simulink model "Car24withDspace"  (R2024a)
settings: Solver=FixedStepAuto  StartTime=0.0  StopTime=Inf  FixedStep=0.001  RelTol=1e-3
PostLoadFcn:
  | if any(exist('dsrtsu_mdlpostloadfcn', 'file') ~= 0), dsrtsu_mdlpostloadfcn('Execute', bdroot); end
InitFcn:
  | , if any(exist('dsmpb_private', 'file') ~= 0), dsmpb_private('dsmpb_mdlclblib', 'Init', bdroot); end,
model workspace (MAT data in the model file):
  indicator = -1
libraries: dsmpblib x8
PreSaveFcn:
  | , if any(exist('dsmpb_private', 'file') ~= 0), dsmpb_private('dsmpb_mdlclblib', 'PreSave', bdroot); end,
CloseFcn:
  | , if any(exist('dsmpb_private', 'file') ~= 0), dsmpb_private('dsmpb_mdlclblib', 'Close', bdroot); end,
settings Model: DSMPB_ID_DATA={'798',struct('BlockId','ba278ee5-6691-4485-94d8-efd942a21a20','SignalIds',{{'fcd8faac-c2ce-41ea-aead-0dfdf2c47ef0'}}),'799',struct('BlockId','a8e41c90-77fc-4f06-b46f-94a13d6c991a','SignalIds',{{'22f08aa9-6fcd-41a1-b62d-e962f18854da'}}),'800',struct('BlockId','31fcda0f-fd6e-4941-ae8a-2ba19cb6e7f7','SignalIds',{{'35c98d34-17e7-4115-963b-beec5af4cec8'}}),'801',struct('BlockId','201071ae-2b6e-446e-b4ec-6a6734ee09dc','SignalIds',{{'1d100d76-8f1b-4c24-9a3c-279a1ced5831'}}),'802',struct('BlockId','a6d9fb5c-79d9-4b84-be40-f4d025ad3cea','SignalIds',{{'1cd988e0-b042-4718-91dc-4e913c3a45d9'}}),'803',struct('BlockId','53d4ca67-4f96-4e4a-b985-d2b7837ee7a0','SignalIds',{{'230ce85a-856b-4b55-a826-97e40144e857'}}),'804',struct('BlockId','a190365b-236b-46d3-8d77-caf955faebcf','SignalIds',{{'146f610b-4436-47f4-bba7-306650b5bba2'}}),'805',struct('BlockId','8fdb49cd-8d95-41ce-94e1-bab524caa5ea','SignalIds',{{'c30a0cdc-fc87-413d-a2e7-a08f688cb26a'}})}  Creator=thipp  LastModifiedBy=thipp
settings SolverCC: AutoInsertRateTranBlk=on
settings OptimizationCC: BlockReduction=off  ConditionallyExecuteInputs=off  OptimizeBlockIOStorage=off  BufferReuse=off  EnhancedBackFolding=on  PassReuseOutputArgsThreshold=0  MaxStackSize=64  OptimizeBlockOrder=speed  DifferentSizesBufferReuse=on
settings DebuggingCC: TasksWithSamePriorityMsg=none  ParameterTunabilityLossMsg=error
settings HardwareCC: ProdBitPerLong=64  ProdLargestAtomicInteger=Integer  ProdWordSize=32  ProdLongLongMode=on  ProdHWDeviceType=Custom Processor->Custom  UseEmbeddedCoderFeatures=off  UseSimulinkCoderFeatures=off
settings ModelReferenceCC: EnableParallelModelReferenceBuilds=on
settings SFSimCC: MATLABDynamicMemAlloc=off
settings RTWCC: Description=dSPACE Target DSRT - Generates SIC files for import by ConfigurationDesk and VEOS. Provides code generation for Simulink models imported in ConfigurationDesk.  SystemTargetFile=dsrt.tlc  GenCodeOnly=on  MakeCommand=make_dsrt  TemplateMakefile=dsrt_default_tmf  RTWVerbose=off  BuildConfiguration=Faster Runs
settings CodeAppCC: ForceParamTrailComments=on  OperatorAnnotations=on
settings STFCustomTargetCC: TargetLangStandard=C89/C90 (ANSI)  ParMdlRefBuildCompliant=on  GRTInterface=off  UseToolchainInfoCompliant=off  SystemTargetFile=dsrt.tlc
settings GRTTargetCC: TargetLangStandard=C89/C90 (ANSI)  CompOptLevelCompliant=off  ConcurrentExecutionCompliant=off  CombineOutputUpdateFcns=off  MatFileLogging=off  CPPClassGenCompliant=off  UseToolchainInfoCompliant=off

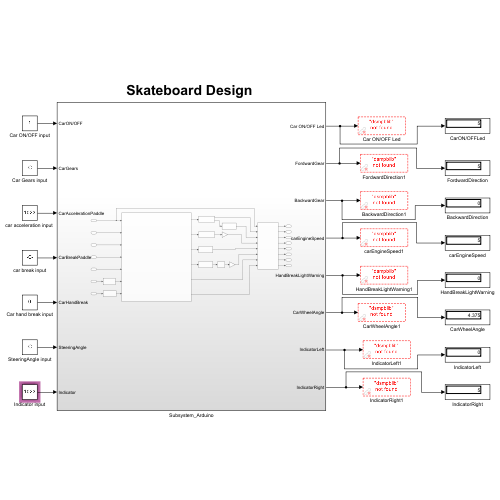
[thumbnail: Simulink's stored preview of the top-level diagram]
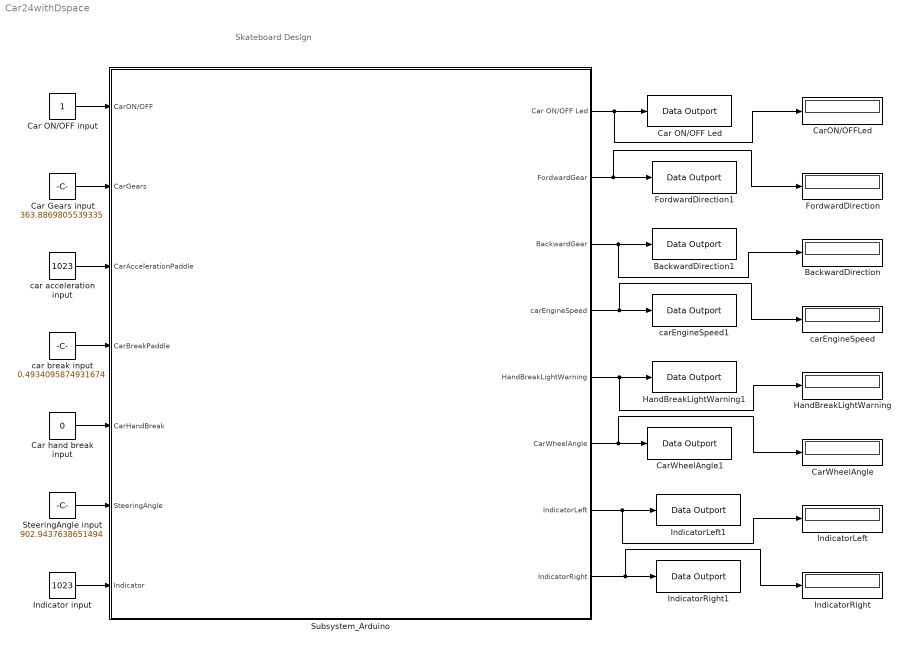
== system Car24withDspace ==
  note: Skateboard Design
  BackwardDirection : Display
  BackwardDirection1 : dsmpblib/Data Outport  Priority=-10000
      settings: SourceProductName=dSPACE Model Interface Package for Simulink (MIPS)
  Car Gears input : Constant  Value=363.8869805539335
  Car ON/OFF Led : dsmpblib/Data Outport  Priority=-10000
      settings: SourceProductName=dSPACE Model Interface Package for Simulink (MIPS)
  Car ON/OFF input : Constant
  Car hand break input : Constant  Value=0
  CarON/OFFLed : Display
  CarWheelAngle : Display
  CarWheelAngle1 : dsmpblib/Data Outport  Priority=-10000
      settings: SourceProductName=dSPACE Model Interface Package for Simulink (MIPS)
  FordwardDirection : Display
  FordwardDirection1 : dsmpblib/Data Outport  Priority=-10000
      settings: SourceProductName=dSPACE Model Interface Package for Simulink (MIPS)
  HandBreakLightWarning : Display
  HandBreakLightWarning1 : dsmpblib/Data Outport  Priority=-10000
      settings: SourceProductName=dSPACE Model Interface Package for Simulink (MIPS)
  Indicator input : Constant  Value=1023
  IndicatorLeft : Display
  IndicatorLeft1 : dsmpblib/Data Outport  Priority=-10000
      settings: SourceProductName=dSPACE Model Interface Package for Simulink (MIPS)
  IndicatorRight : Display
  IndicatorRight1 : dsmpblib/Data Outport  Priority=-10000
      settings: SourceProductName=dSPACE Model Interface Package for Simulink (MIPS)
  SteeringAngle input : Constant  Value=902.9437638651494
  Subsystem_Arduino : Subsystem
  "car acceleration input " : Constant  Value=1023
  car break input : Constant  Value=0.4934095874931674
  carEngineSpeed : Display
  carEngineSpeed1 : dsmpblib/Data Outport  Priority=-10000
      settings: SourceProductName=dSPACE Model Interface Package for Simulink (MIPS)
  wires:
  Subsystem_Arduino/3(BackwardGear) -> BackwardDirection1/1, BackwardDirection/1
  Subsystem_Arduino/4(carEngineSpeed) -> carEngineSpeed1/1, carEngineSpeed/1
  Subsystem_Arduino/5(HandBreakLightWarning) -> HandBreakLightWarning1/1, HandBreakLightWarning/1
  Subsystem_Arduino/6(CarWheelAngle) -> CarWheelAngle1/1, CarWheelAngle/1
  Subsystem_Arduino/7(IndicatorLeft) -> IndicatorLeft1/1, IndicatorLeft/1
  Subsystem_Arduino/8(IndicatorRight) -> IndicatorRight1/1, IndicatorRight/1
  Subsystem_Arduino/1(Car ON/OFF Led) -> Car ON/OFF Led/1, CarON/OFFLed/1
  Car Gears input/1 -> Subsystem_Arduino/2(CarGears)
  car break input/1 -> Subsystem_Arduino/4(CarBreakPaddle)
  SteeringAngle input/1 -> Subsystem_Arduino/6(SteeringAngle)
  Car ON/OFF input/1 -> Subsystem_Arduino/1(CarON/OFF)
  Car hand break input/1 -> Subsystem_Arduino/5("CarHandBreak ")
  Indicator input/1 -> Subsystem_Arduino/7(Indicator)
  "car acceleration input "/1 -> Subsystem_Arduino/3(CarAccelerationPaddle)
  Subsystem_Arduino/2(FordwardGear) -> FordwardDirection1/1, FordwardDirection/1

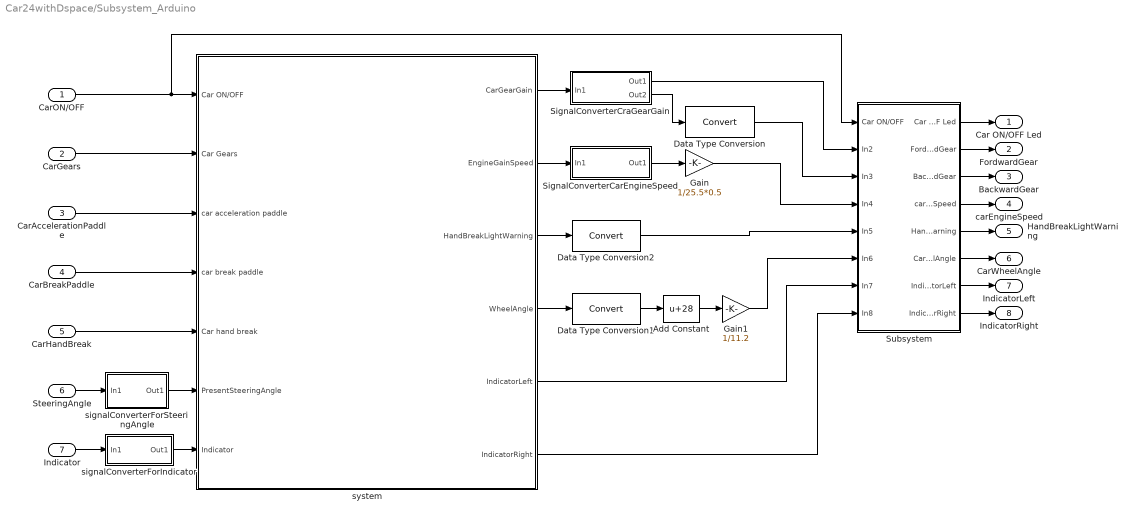
== system Car24withDspace/Subsystem_Arduino ==
  CarON/OFF : Inport
  CarGears : Inport  Port=2
  CarAccelerationPaddle : Inport  Port=3
  CarBreakPaddle : Inport  Port=4
  "CarHandBreak " : Inport  Port=5
  SteeringAngle : Inport  Port=6
  Indicator : Inport  Port=7
  Add Constant : Bias  Bias=28  SaturateOnIntegerOverflow=off
  Data Type Conversion : DataTypeConversion  SaturateOnIntegerOverflow=off  RndMeth=Floor
  Data Type Conversion1 : DataTypeConversion  SaturateOnIntegerOverflow=off  RndMeth=Floor
  Data Type Conversion2 : DataTypeConversion  SaturateOnIntegerOverflow=off  RndMeth=Floor
  Gain : Gain  Gain=1/25.5*0.5
  Gain1 : Gain  Gain=1/11.2
  SignalConverterCarEngineSpeed : Subsystem
  SignalConverterCraGearGain : Subsystem
  Subsystem : Subsystem
  signalConverterForIndicator : Subsystem
  signalConverterForSteeringAngle : Subsystem
  system : Subsystem
  Car ON/OFF Led : Outport
  FordwardGear : Outport  Port=2
  BackwardGear : Outport  Port=3
  carEngineSpeed : Outport  Port=4
  HandBreakLightWarning : Outport  Port=5
  CarWheelAngle : Outport  Port=6
  IndicatorLeft : Outport  Port=7
  IndicatorRight : Outport  Port=8
  wires:
  CarBreakPaddle/1 -> system/4(car break paddle)
  CarAccelerationPaddle/1 -> system/3(car acceleration paddle)
  "CarHandBreak "/1 -> system/5("Car hand break ")
  CarGears/1 -> system/2(Car Gears)
  CarON/OFF/1 -> Subsystem/1(Car ON/OFF), system/1(Car ON/OFF)
  SteeringAngle/1 -> signalConverterForSteeringAngle/1(In1)
  signalConverterForSteeringAngle/1(Out1) -> system/6(PresentSteeringAngle)
  Indicator/1 -> signalConverterForIndicator/1(In1)
  signalConverterForIndicator/1(Out1) -> system/7(Indicator)
  system/2(EngineGainSpeed) -> SignalConverterCarEngineSpeed/1(In1)
  system/1(CarGearGain) -> SignalConverterCraGearGain/1(In1)
  SignalConverterCraGearGain/2(Out2) -> Data Type Conversion/1
  system/4(WheelAngle) -> Data Type Conversion1/1
  system/3(HandBreakLightWarning) -> Data Type Conversion2/1
  SignalConverterCarEngineSpeed/1(Out1) -> Gain/1
  Data Type Conversion1/1 -> Add Constant/1
  Add Constant/1 -> Gain1/1
  Data Type Conversion/1 -> Subsystem/3(In3)
  Gain/1 -> Subsystem/4(In4)
  Data Type Conversion2/1 -> Subsystem/5(In5)
  Gain1/1 -> Subsystem/6(In6)
  system/5(IndicatorLeft) -> Subsystem/7(In7)
  system/6(IndicatorRight) -> Subsystem/8(In8)
  Subsystem/1(Car ON/OFF Led) -> Car ON/OFF Led/1
  Subsystem/2(FordwardGear) -> FordwardGear/1
  Subsystem/3(BackwardGear) -> BackwardGear/1
  Subsystem/4(carEngineSpeed) -> carEngineSpeed/1
  Subsystem/5(HandBreakLightWarning) -> HandBreakLightWarning/1
  Subsystem/6(CarWheelAngle) -> CarWheelAngle/1
  Subsystem/7(IndicatorLeft) -> IndicatorLeft/1
  Subsystem/8(IndicatorRight) -> IndicatorRight/1
  SignalConverterCraGearGain/1(Out1) -> Subsystem/2(In2)

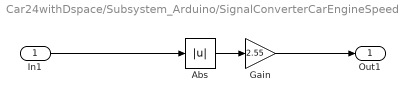
== system Car24withDspace/Subsystem_Arduino/SignalConverterCarEngineSpeed ==
  In1 : Inport
  Abs : Abs  SaturateOnIntegerOverflow=off
  Gain : Gain  Gain=2.55
  Out1 : Outport
  wires:
  Abs/1 -> Gain/1
  Gain/1 -> Out1/1
  In1/1 -> Abs/1

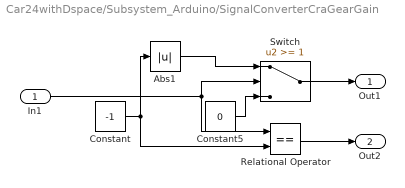
== system Car24withDspace/Subsystem_Arduino/SignalConverterCraGearGain ==
  In1 : Inport
  Abs1 : Abs  SaturateOnIntegerOverflow=off
  Constant : Constant  Value=-1
  Constant5 : Constant  Value=0
  Relational Operator : RelationalOperator  Operator===  OutDataTypeStr=boolean  RndMeth=Simplest  InputSameDT=off
  Switch : Switch  Threshold=1  SaturateOnIntegerOverflow=off  InputSameDT=off
  Out1 : Outport
  Out2 : Outport  Port=2
  wires:
  Switch/1 -> Out1/1
  Abs1/1 -> Switch/1
  Constant5/1 -> Switch/3
  Constant/1 -> Relational Operator/2, Abs1/1
  In1/1 -> Relational Operator/1, Switch/2
  Relational Operator/1 -> Out2/1

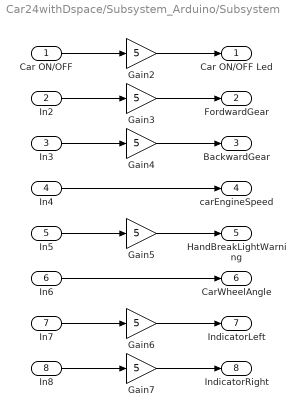
== system Car24withDspace/Subsystem_Arduino/Subsystem ==
  Car ON/OFF : Inport
  In2 : Inport  Port=2
  In3 : Inport  Port=3
  In4 : Inport  Port=4
  In5 : Inport  Port=5
  In6 : Inport  Port=6
  In7 : Inport  Port=7
  In8 : Inport  Port=8
  Gain{2..7} (6 alike) : Gain  Gain=5
  Car ON/OFF Led : Outport
  FordwardGear : Outport  Port=2
  BackwardGear : Outport  Port=3
  carEngineSpeed : Outport  Port=4
  HandBreakLightWarning : Outport  Port=5
  CarWheelAngle : Outport  Port=6
  IndicatorLeft : Outport  Port=7
  IndicatorRight : Outport  Port=8
  wires:
  In6/1 -> CarWheelAngle/1
  In4/1 -> carEngineSpeed/1
  Gain3/1 -> FordwardGear/1
  Gain7/1 -> IndicatorRight/1
  Gain5/1 -> HandBreakLightWarning/1
  In5/1 -> Gain5/1
  Gain4/1 -> BackwardGear/1
  Gain6/1 -> IndicatorLeft/1
  Gain2/1 -> Car ON/OFF Led/1
  In3/1 -> Gain4/1
  In7/1 -> Gain6/1
  In8/1 -> Gain7/1
  In2/1 -> Gain3/1
  Car ON/OFF/1 -> Gain2/1

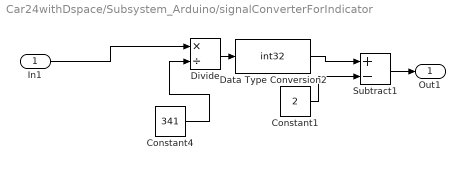
== system Car24withDspace/Subsystem_Arduino/signalConverterForIndicator ==
  In1 : Inport
  Constant1 : Constant  Value=2
  Constant4 : Constant  Value=341
  Data Type Conversion2 : DataTypeConversion  OutDataTypeStr=int32  ConvertRealWorld=Stored Integer (SI)  RndMeth=Ceiling  SaturateOnIntegerOverflow=off
  Divide : Product  Inputs=*/
  Subtract1 : Sum  Inputs=+-
  Out1 : Outport
  wires:
  Constant4/1 -> Divide/2
  Data Type Conversion2/1 -> Subtract1/1
  Divide/1 -> Data Type Conversion2/1
  Subtract1/1 -> Out1/1
  Constant1/1 -> Subtract1/2
  In1/1 -> Divide/1

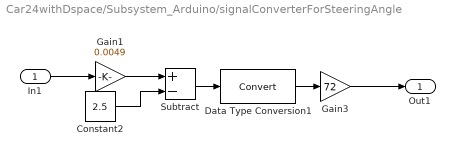
== system Car24withDspace/Subsystem_Arduino/signalConverterForSteeringAngle ==
  In1 : Inport
  Constant2 : Constant  Value=2.5
  Data Type Conversion1 : DataTypeConversion  SaturateOnIntegerOverflow=off  RndMeth=Floor
  Gain1 : Gain  Gain=0.0049
  Gain3 : Gain  Gain=72
  Subtract : Sum  Inputs=+-
  Out1 : Outport
  wires:
  Gain1/1 -> Subtract/1
  Constant2/1 -> Subtract/2
  Subtract/1 -> Data Type Conversion1/1
  Gain3/1 -> Out1/1
  In1/1 -> Gain1/1
  Data Type Conversion1/1 -> Gain3/1

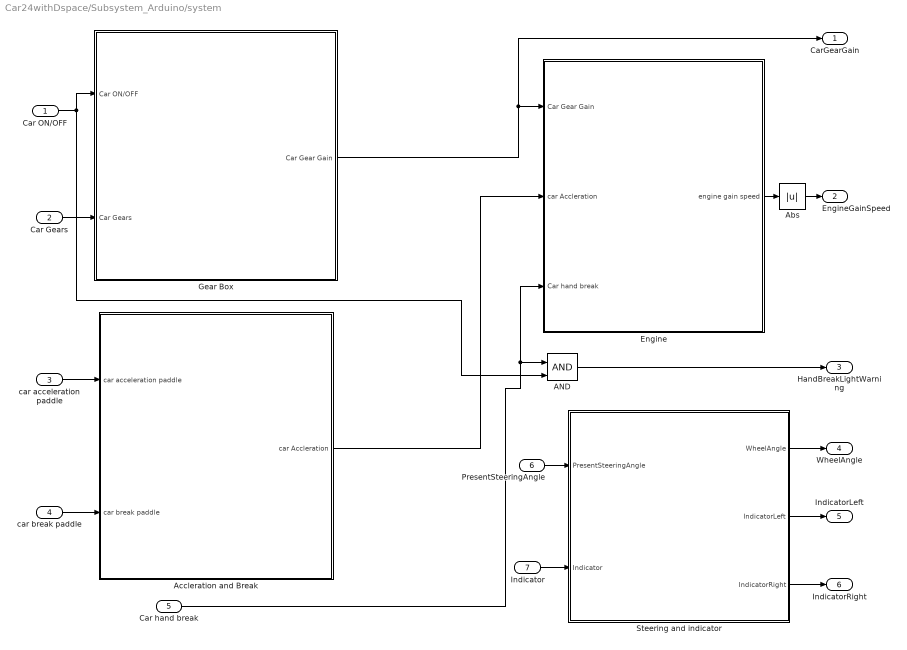
== system Car24withDspace/Subsystem_Arduino/system ==
  Car ON/OFF : Inport
  Car Gears : Inport  Port=2
  car acceleration paddle : Inport  Port=3
  car break paddle : Inport  Port=4
  "Car hand break " : Inport  Port=5
  PresentSteeringAngle : Inport  Port=6
  Indicator : Inport  Port=7
  AND : Logic  IconShape=distinctive  AllPortsSameDT=off  OutDataTypeStr=boolean
  Abs : Abs  SaturateOnIntegerOverflow=off
  Accleration and Break : Subsystem
  Engine : Subsystem
  Gear Box : Subsystem
  "Steering and indicator " : Subsystem
  CarGearGain : Outport
  EngineGainSpeed : Outport  Port=2
  HandBreakLightWarning : Outport  Port=3
  WheelAngle : Outport  Port=4
  IndicatorLeft : Outport  Port=5
  IndicatorRight : Outport  Port=6
  wires:
  Car ON/OFF/1 -> Gear Box/1(Car ON/OFF), AND/2
  Accleration and Break/1(car Accleration) -> Engine/2(car Accleration)
  "Steering and indicator "/3(IndicatorRight) -> IndicatorRight/1
  "Steering and indicator "/2(IndicatorLeft) -> IndicatorLeft/1
  car acceleration paddle/1 -> Accleration and Break/1(car acceleration paddle)
  Indicator/1 -> "Steering and indicator "/2(Indicator)
  "Car hand break "/1 -> Engine/3("Car hand break "), AND/1
  Engine/1(engine gain speed) -> Abs/1
  car break paddle/1 -> Accleration and Break/2(car break paddle)
  Car Gears/1 -> Gear Box/2(Car Gears)
  Abs/1 -> EngineGainSpeed/1
  "Steering and indicator "/1(WheelAngle) -> WheelAngle/1
  AND/1 -> HandBreakLightWarning/1
  PresentSteeringAngle/1 -> "Steering and indicator "/1(PresentSteeringAngle)
  Gear Box/1(Car Gear Gain) -> CarGearGain/1, Engine/1(Car Gear Gain)

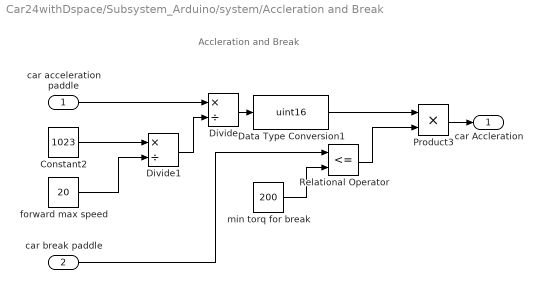
== system Car24withDspace/Subsystem_Arduino/system/Accleration and Break ==
  note: Accleration and Break
  car acceleration paddle : Inport
  car break paddle : Inport  Port=2
  Constant2 : Constant  Value=1023
  Data Type Conversion1 : DataTypeConversion  OutDataTypeStr=uint16  SaturateOnIntegerOverflow=off  RndMeth=Floor
  Divide : Product  Inputs=*/  RndMeth=Zero  SaturateOnIntegerOverflow=on
  Divide1 : Product  Inputs=*/  RndMeth=Zero  SaturateOnIntegerOverflow=on
  Product3 : Product
  Relational Operator : RelationalOperator  Operator=<=  OutDataTypeStr=boolean  RndMeth=Simplest  InputSameDT=off
  forward max speed : Constant  Value=20
  min torq for break : Constant  Value=200
  car Accleration : Outport
  wires:
  min torq for break/1 -> Relational Operator/2
  Divide/1 -> Data Type Conversion1/1
  forward max speed/1 -> Divide1/2
  car break paddle/1 -> Relational Operator/1
  Data Type Conversion1/1 -> Product3/1
  Constant2/1 -> Divide1/1
  Divide1/1 -> Divide/2
  Relational Operator/1 -> Product3/2
  car acceleration paddle/1 -> Divide/1
  Product3/1 -> car Accleration/1

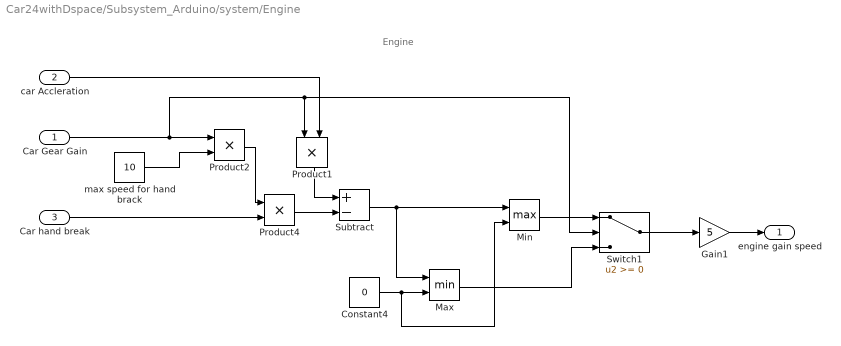
== system Car24withDspace/Subsystem_Arduino/system/Engine ==
  note: Engine
  Car Gear Gain : Inport
  car Accleration : Inport  Port=2
  "Car hand break " : Inport  Port=3
  Constant4 : Constant  Value=0
  Gain1 : Gain  Gain=5
  Max : MinMax  Inputs=2
  Min : MinMax  Function=max  Inputs=2
  Product1 : Product
  Product2 : Product
  Product4 : Product
  Subtract : Sum  Inputs=+-
  Switch1 : Switch  SaturateOnIntegerOverflow=off  InputSameDT=off
  max speed for hand brack : Constant  Value=10
  engine gain speed : Outport
  wires:
  Subtract/1 -> Min/1, Max/1
  Switch1/1 -> Gain1/1
  Product2/1 -> Product4/1
  Product1/1 -> Subtract/1
  Product4/1 -> Subtract/2
  Constant4/1 -> Min/2, Max/2
  max speed for hand brack/1 -> Product2/2
  Car Gear Gain/1 -> Product1/1, Switch1/2, Product2/1
  Max/1 -> Switch1/3
  Min/1 -> Switch1/1
  car Accleration/1 -> Product1/2
  "Car hand break "/1 -> Product4/2
  Gain1/1 -> engine gain speed/1

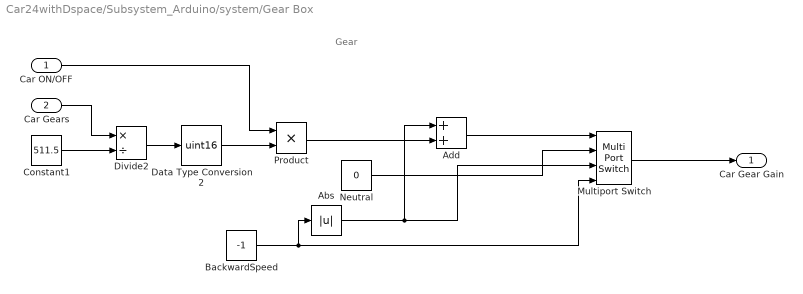
== system Car24withDspace/Subsystem_Arduino/system/Gear Box ==
  note: Gear
  Car ON/OFF : Inport
  Car Gears : Inport  Port=2
  Abs : Abs  SaturateOnIntegerOverflow=off
  Add : Sum
  BackwardSpeed : Constant  Value=-1
  Constant1 : Constant  Value=511.5
  Data Type Conversion2 : DataTypeConversion  OutDataTypeStr=uint16  RndMeth=Nearest  SaturateOnIntegerOverflow=off
  Divide2 : Product  Inputs=*/  RndMeth=Zero  SaturateOnIntegerOverflow=on
  Multiport Switch : MultiPortSwitch  SaturateOnIntegerOverflow=off  InputSameDT=off
  Neutral : Constant  Value=0
  Product : Product
  Car Gear Gain : Outport
  wires:
  Add/1 -> Multiport Switch/1
  Neutral/1 -> Multiport Switch/2
  Constant1/1 -> Divide2/2
  Product/1 -> Add/2
  BackwardSpeed/1 -> Abs/1, Multiport Switch/4
  Data Type Conversion2/1 -> Product/2
  Divide2/1 -> Data Type Conversion2/1
  Abs/1 -> Add/1, Multiport Switch/3
  Multiport Switch/1 -> Car Gear Gain/1
  Car ON/OFF/1 -> Product/1
  Car Gears/1 -> Divide2/1

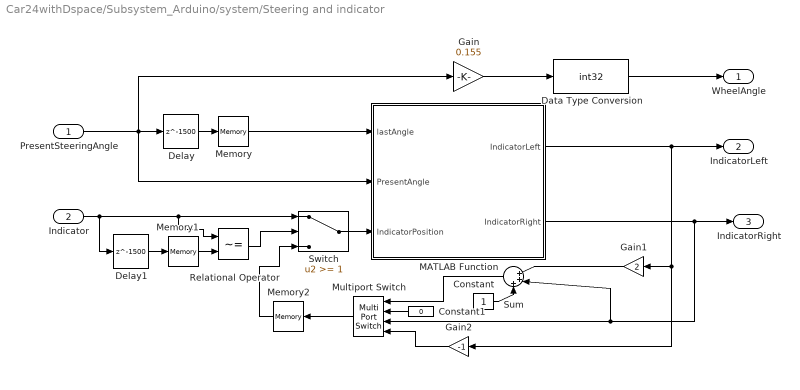
== system Car24withDspace/Subsystem_Arduino/system/Steering and indicator  ==
  PresentSteeringAngle : Inport
  Indicator : Inport  Port=2
  Constant : Constant
  Constant1 : Constant  Value=0
  Data Type Conversion : DataTypeConversion  OutDataTypeStr=int32  SaturateOnIntegerOverflow=off  RndMeth=Floor
  Delay : Delay  DelayLength=1500
  Delay1 : Delay  DelayLength=1500
  Gain : Gain  Gain=0.155
  Gain1 : Gain  Gain=2
  Gain2 : Gain  Gain=-1
  MATLAB Function : MATLAB Function  TreatAsAtomicUnit=on
  Memory : Memory
  Memory1 : Memory
  Memory2 : Memory
  Multiport Switch : MultiPortSwitch  SaturateOnIntegerOverflow=off  InputSameDT=off
  Relational Operator : RelationalOperator  Operator=~=  OutDataTypeStr=boolean  RndMeth=Simplest  InputSameDT=off
  Sum : Sum  Inputs=|+++
  Switch : Switch  Threshold=1  SaturateOnIntegerOverflow=off  InputSameDT=off
  WheelAngle : Outport
  IndicatorLeft : Outport  Port=2
  IndicatorRight : Outport  Port=3
  wires:
  PresentSteeringAngle/1 -> MATLAB Function/2(PresentAngle), Gain/1, Delay/1
  MATLAB Function/1(IndicatorLeft) -> Gain2/1, Gain1/1, IndicatorLeft/1
  Memory/1 -> MATLAB Function/1(lastAngle)
  Delay/1 -> Memory/1
  Indicator/1 -> Delay1/1, Relational Operator/1, Switch/1
  Relational Operator/1 -> Switch/2
  Switch/1 -> MATLAB Function/3(IndicatorPosition)
  Memory1/1 -> Relational Operator/2
  Delay1/1 -> Memory1/1
  Memory2/1 -> Switch/3
  Sum/1 -> Multiport Switch/1
  Constant/1 -> Sum/3
  Constant1/1 -> Multiport Switch/2
  MATLAB Function/2(IndicatorRight) -> IndicatorRight/1, Sum/2, Multiport Switch/3
  Gain1/1 -> Sum/1
  Gain2/1 -> Multiport Switch/4
  Multiport Switch/1 -> Memory2/1
  Gain/1 -> Data Type Conversion/1
  Data Type Conversion/1 -> WheelAngle/1

== matlab function Car24withDspace/Subsystem_Arduino/system/Steering and indicator /MATLAB Function ==
  data: IndicatorLeft output; IndicatorRight output; lastAngle input; PresentAngle input; IndicatorPosition input
function [IndicatorLeft, IndicatorRight] = fcn(lastAngle, PresentAngle, IndicatorPosition)
    % Determine the turning direction
    turning = 0;
    if PresentAngle> lastAngle 
        turning = 1; % Turning right
    elseif PresentAngle< lastAngle 
        turning = -1; % Turning left
    end
    
    % Update the indicator position based on the turning direction
    if IndicatorPosition == 1 && turning == -1
        IndicatorPosition = 0; % Cancel right indicator when turning left
    elseif IndicatorPosition == -1 && turning == 1
        IndicatorPosition = 0; % Cancel left indicator when turning right
    end
    
    % Determine the state of left and right indicators
    if IndicatorPosition == -1
        IndicatorLeft = 1; % Left indicator is on
    else
        IndicatorLeft = 0;
    end
    if IndicatorPosition == 1
        IndicatorRight = 1; % Right indicator is on
    else
        IndicatorRight = 0;
    end
end
